simulink model "slexHARAndroidExample"  (R2021a)
settings: Solver=FixedStepAuto  StartTime=0.0  StopTime=10.0  RelTol=1e-3
model workspace (MAT data in the model file):
  jumpingImg = [255 255 255 255 255 255 255 255 255 255 255 255 ... (960000 elements, 800x400x3)]
  runningImg = [255 255 255 255 255 255 255 255 255 255 255 255 ... (960000 elements, 800x400x3)]
  sittingImg = [255 255 255 255 255 255 255 255 255 255 255 255 ... (960000 elements, 800x400x3)]
  standingImg = [255 255 255 255 255 255 255 255 255 255 255 255 ... (960000 elements, 800x400x3)]
  walkingImg = [255 255 255 255 255 255 255 255 255 255 255 255 ... (960000 elements, 800x400x3)]
undefined symbols (not defined in the file or in its folder): Acc_X, Acc_Y, Acc_Z, HARAndroidModel, Predicted_Activity
libraries: androiduilib x4, androidsensorlib x1, androidaudiovideolib x1
(part 1 of 2)
settings Model: Creator=The MathWorks, Inc.  LastModifiedBy=The MathWorks, Inc.
settings SolverCC: AlgebraicLoopSolver=TrustRegion  DecoupledContinuousIntegration=on
settings DataIOCC: ReturnWorkspaceOutputs=off
settings OptimizationCC: EnhancedBackFolding=on  StrengthReduction=on  PassReuseOutputArgsAs=Individual arguments  MaxStackSize=64  OptimizeBlockOrder=speed  DifferentSizesBufferReuse=on  EfficientTunableParamExpr=on
settings DebuggingCC: ParameterTunabilityLossMsg=error  SFMachineParentedDataDiag=warning  ArithmeticOperatorsInVariantConditions=warning
settings HardwareCC: ProdBitPerPointer=32  ProdBitPerSizeT=32  ProdBitPerPtrDiffT=32  ProdLargestAtomicInteger=Long  ProdLargestAtomicFloat=Double  ProdWordSize=32  ProdHWDeviceType=ARM Compatible->ARM Cortex
settings SFSimCC: SimUseLocalCustomCode=off  MATLABDynamicMemAlloc=off
settings RTWCC: SystemTargetFile=ert.tlc  HardwareBoard=Android Device  TLCOptions="-aInlineSetEventsForThisBaseRateFcn=TLC_FALSE -aSuppressMultiTaskScheduler=TLC_FALSE  -aRateBasedStepFcn=0"  TemplateMakefile=ert_default_tmf  GenerateReport=on  RTWUseLocalCustomCode=off  Toolchain=Android SDK/NDK Tools  BuildConfiguration=Faster Runs  IncludeHyperlinkInReport=on  LaunchReport=on  GenerateTraceInfo=on  GenerateTraceReport=on  GenerateTraceReportSl=on  GenerateTraceReportSf=on  GenerateTraceReportEml=on
settings CodeAppCC: ForceParamTrailComments=on  IgnoreCustomStorageClasses=off  OperatorAnnotations=on  SimulinkDataObjDesc=on  SFDataObjDesc=on  InsertBlockDesc=on
settings ERTTargetCC: SupportVariableSizeSignals=on

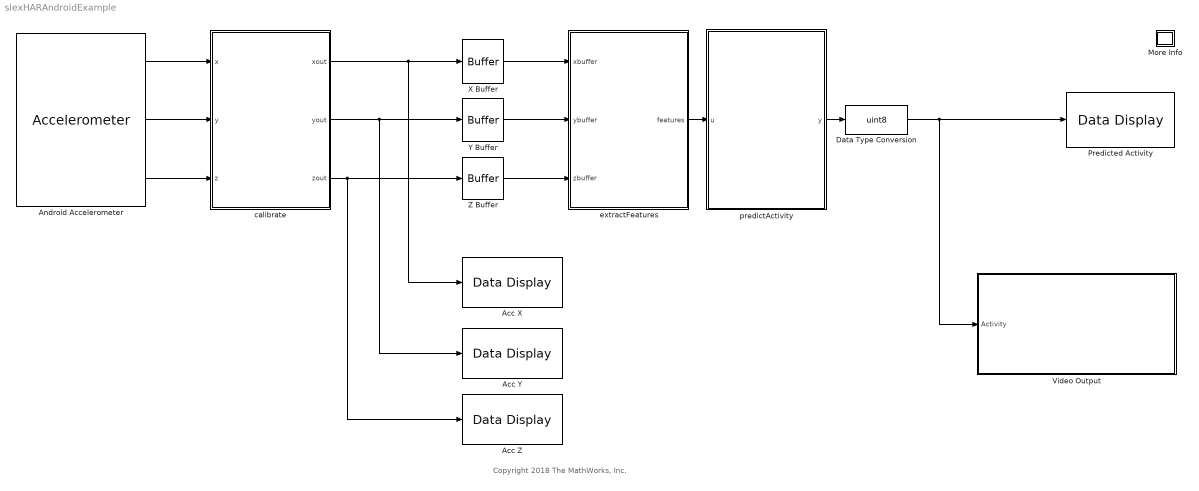
== system slexHARAndroidExample ==
  note: Copyright 2018 The MathWorks, Inc.
  Acc X : androiduilib/Data Display  DataDisplayId=HARAndroidModel/Acc_X  Format=Float  Precision=6  SimulateUsing=Code generation  blockPlatform=Android
      settings: SourceProductBaseCode=ANDROID
  Acc Y : androiduilib/Data Display  DataDisplayId=HARAndroidModel/Acc_Y  Format=Float  Precision=6  SimulateUsing=Code generation  blockPlatform=Android
      settings: SourceProductBaseCode=ANDROID
  Acc Z : androiduilib/Data Display  DataDisplayId=HARAndroidModel/Acc_Z  Format=Float  Precision=6  SimulateUsing=Code generation  blockPlatform=Android
      settings: SourceProductBaseCode=ANDROID
  Android Accelerometer : androidsensorlib/Accelerometer  OutputVector=off  SampleTime=0.1  BlockPlatform=Android
      settings: SourceProductBaseCode=ANDROID
  Data Type Conversion : DataTypeConversion  OutDataTypeStr=uint8
  More Info : Subsystem
      settings: OpenFcn=showExample('stats/HARDeploymentExample')
      mask Display: disp('?')
  Predicted Activity : androiduilib/Data Display  DataDisplayId=HARAndroidModel/Predicted_Activity  Format=Float  Precision=6  SimulateUsing=Code generation  blockPlatform=Android
      settings: SourceProductBaseCode=ANDROID
  Video Output : Subsystem
  X Buffer : Buffer  N=32  V=12  OutputFrames=off
  Y Buffer : Buffer  N=32  V=12  OutputFrames=off
  Z Buffer : Buffer  N=32  V=12  OutputFrames=off
  calibrate : MATLAB Function  TreatAsAtomicUnit=on
  extractFeatures : MATLAB Function  TreatAsAtomicUnit=on
  predictActivity : MATLAB Function  TreatAsAtomicUnit=on
  wires:
  Data Type Conversion/1 -> Video Output/1(Activity), Predicted Activity/1
  calibrate/3(zout) -> Acc Z/1, Z Buffer/1
  Y Buffer/1 -> extractFeatures/2(ybuffer)
  Android Accelerometer/2 -> calibrate/2(y)
  extractFeatures/1(features) -> predictActivity/1(u)
  X Buffer/1 -> extractFeatures/1(xbuffer)
  Android Accelerometer/3 -> calibrate/3(z)
  calibrate/2(yout) -> Acc Y/1, Y Buffer/1
  predictActivity/1(y) -> Data Type Conversion/1
  Z Buffer/1 -> extractFeatures/3(zbuffer)
  calibrate/1(xout) -> Acc X/1, X Buffer/1
  Android Accelerometer/1 -> calibrate/1(x)
